simulink model "p6"  (R2015a)
settings: Solver=ode3  StartTime=0.0  StopTime=simtime  FixedStep=step  RelTol=1e-3
values from neighbouring files (symbols this model uses):
  A = [ 0 1 ; (1/J)*(g*a-k) -beta/J ]    [lab3.m]
  B = [ 0 ; 1/J ]    [lab3.m]
  C = [ 1 0 ; 0 1 ]    [lab3.m]
  cinit = [ pi/4 ; 0 ]    [lab3.m]
  D = [ 0 ; 0 ]    [lab3.m]
settings Model: Creator=Pedro  LastModifiedBy=Pedro

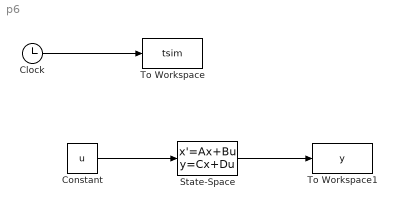
== system p6 ==
  Clock : Clock
  Constant : Constant  Value=u
  State-Space : StateSpace  A=A  B=B  C=C  D=D  X0=cinit
  To Workspace : ToWorkspace  VariableName=tsim  SampleTime=-1
  To Workspace1 : ToWorkspace  VariableName=y  SampleTime=-1
  wires:
  Clock/1 -> To Workspace/1
  Constant/1 -> State-Space/1
  State-Space/1 -> To Workspace1/1
